simulink model "Single_String_with_shufflingconverters"  (R2019a)
settings: Solver=FixedStepDiscrete  StartTime=0.0  StopTime=0.2  RelTol=1e-3
libraries: powerlib x24, re_lib x4
settings Model: Creator=burge  LastModifiedBy=natha
settings DataIOCC: SaveState=on  ReturnWorkspaceOutputs=off
settings DebuggingCC: PregeneratedLibrarySubsystemCodeDiagnostic=none  ArithmeticOperatorsInVariantConditions=warning
settings SFSimCC: SimUseLocalCustomCode=off
settings RTWCC: RTWUseLocalCustomCode=off

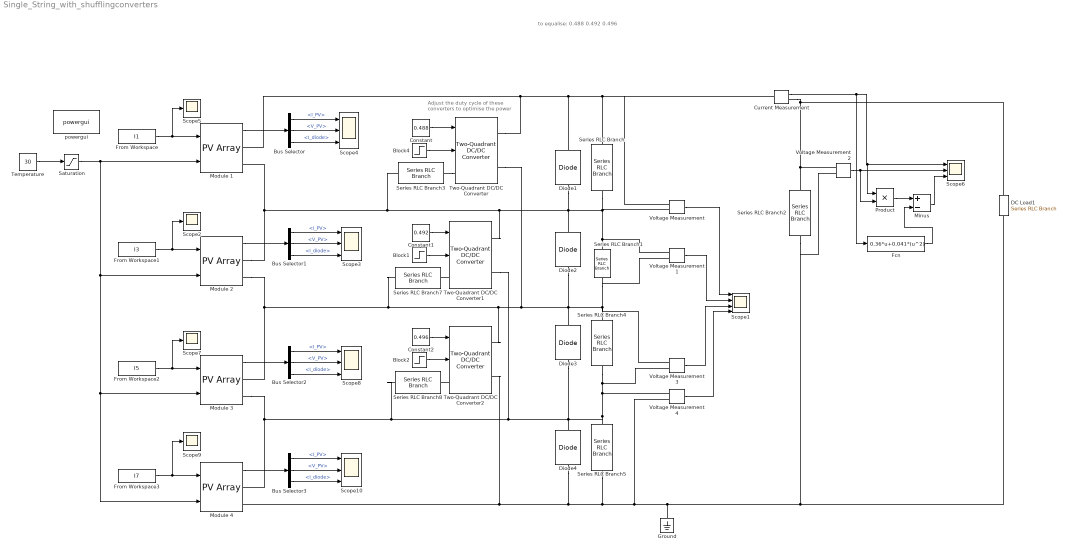
== system Single_String_with_shufflingconverters ==
  note: Adjust the duty cycle of these converters to optimise the power
  note: to equalise:
      | 0.488
      | 0.492
      | 0.496
  Block1 : Step  Time=0  Before=1  After=0  SampleTime=5e-5
  Block2 : Step  Time=0  Before=1  After=0  SampleTime=5e-5
  Block4 : Step  Time=0  Before=1  After=0  SampleTime=5e-5
  Bus Selector{,1..3} (4 alike) : BusSelector  OutputSignals=I_PV,V_PV,I_diode
  Constant : Constant  Value=0.488
  Constant1 : Constant  Value=0.492
  Constant2 : Constant  Value=0.496
  Current Measurement : powerlib/Measurements/Current Measurement  PhasorSimulation=off  OutputType=Complex  PSBequivalent=0
      settings: SourceProductName=Simscape Electrical
  DC Load1 : powerlib/Elements/Series RLC Branch  LConnTagsString=__new0  RConnTagsString=__new0  BranchType=R  Resistance=9  Inductance=1e-3  SetiL0=off  InitialCurrent=0  Capacitance=1e-6  Setx0=off  InitialVoltage=0  Measurements=None
      settings: SourceProductName=Simscape Electrical
  Diode{1..4} (4 alike) : powerlib/Power Electronics/Diode  Ron=0.05  Lon=0  Vf=0.7  IC=0  UseSnubber=0  Rs=500  Cs=250e-9  Measurements=off
      settings: SourceProductName=Simscape Electrical
  Fcn : Fcn  Expr=0.36*u+0.041*(u^2)
  From Workspace : FromWorkspace  VariableName=I1  OutDataTypeStr=double  SampleTime=0  OutputAfterFinalValue=Holding final value
  From Workspace1 : FromWorkspace  VariableName=I3  OutDataTypeStr=double  SampleTime=0  OutputAfterFinalValue=Holding final value
  From Workspace2 : FromWorkspace  VariableName=I5  OutDataTypeStr=double  SampleTime=0  OutputAfterFinalValue=Holding final value
  From Workspace3 : FromWorkspace  VariableName=I7  OutDataTypeStr=double  SampleTime=0  OutputAfterFinalValue=Holding final value
  Ground : powerlib/Elements/Ground  LConnTagsString=a
      settings: SourceProductName=Simscape Electrical
  Minus : Sum  Inputs=+-
  Module 1 : re_lib/Solar/PV Array  Npar=1  Nser=5  PlotType=array @ 1000 W/m2 & specified temperatures  S_vec="[ 1000  500  100 ]"  Temp_C_vec="[ 45 25  ]"  ModuleName=User-defined  PlotWhenSelected=off  Pm=3.8912  Ncell=1  Voc=0.727  Isc=6.45  Vm=0.64  Im=6.08  beta_Voc_pc=-0.2393  alpha_Isc_pc=0.045  beta_Voc=-0.0017397  alpha_Isc=0.0029025  IL=6.4807  I0=1.3352e-12  nI=0.96977  Rsh=3.547  Rs=0.00078547  BAL=on  Tc=1e-6  Tfilter=5e-5
      settings: SourceProductName=Simscape Electrical
  Module 2 : re_lib/Solar/PV Array  Npar=1  Nser=10  PlotType=array @ 1000 W/m2 & specified temperatures  S_vec="[ 1000  500  100 ]"  Temp_C_vec="[ 45 25  ]"  ModuleName=User-defined  PlotWhenSelected=off  Pm=3.8912  Ncell=1  Voc=0.727  Isc=6.45  Vm=0.64  Im=6.08  beta_Voc_pc=-0.2393  alpha_Isc_pc=0.045  beta_Voc=-0.0017397  alpha_Isc=0.0029025  IL=6.4807  I0=1.3352e-12  nI=0.96977  Rsh=3.547  Rs=0.00078547  BAL=on  Tc=1e-6  Tfilter=5e-5
      settings: SourceProductName=Simscape Electrical
  Module 3 : re_lib/Solar/PV Array  Npar=1  Nser=10  PlotType=array @ 1000 W/m2 & specified temperatures  S_vec="[ 1000  500  100 ]"  Temp_C_vec="[ 45 25  ]"  ModuleName=User-defined  PlotWhenSelected=off  Pm=3.8912  Ncell=1  Voc=0.727  Isc=6.45  Vm=0.64  Im=6.08  beta_Voc_pc=-0.2393  alpha_Isc_pc=0.045  beta_Voc=-0.0017397  alpha_Isc=0.0029025  IL=6.4807  I0=1.3352e-12  nI=0.96977  Rsh=3.547  Rs=0.00078547  BAL=on  Tc=1e-6  Tfilter=5e-5
      settings: SourceProductName=Simscape Electrical
  Module 4 : re_lib/Solar/PV Array  Npar=1  Nser=10  PlotType=array @ 1000 W/m2 & specified temperatures  S_vec="[ 1000  500  100 ]"  Temp_C_vec="[ 45 25  ]"  ModuleName=User-defined  PlotWhenSelected=off  Pm=3.8912  Ncell=1  Voc=0.727  Isc=6.45  Vm=0.64  Im=6.08  beta_Voc_pc=-0.2393  alpha_Isc_pc=0.045  beta_Voc=-0.0017397  alpha_Isc=0.0029025  IL=6.4807  I0=1.3352e-12  nI=0.96977  Rsh=3.547  Rs=0.00078547  BAL=on  Tc=1e-6  Tfilter=5e-5
      settings: SourceProductName=Simscape Electrical
  Product : Product
  Saturation : Saturate  UpperLimit=55  LowerLimit=5
  Scope1 : Scope  NumInputPorts=4
  Scope{3..4,6,8,10} (5 alike) : Scope  NumInputPorts=3
  Scope{2,5,7,9} (4 alike) : Scope
  Series RLC Branch{,1,4..5} (4 alike) : powerlib/Elements/Series RLC Branch  LConnTagsString=__new0  RConnTagsString=__new0  BranchType=C  Resistance=1  Inductance=1e-3  SetiL0=off  InitialCurrent=0  Capacitance=100e-6  Setx0=off  InitialVoltage=0  Measurements=None
      settings: SourceProductName=Simscape Electrical
  Series RLC Branch2 : powerlib/Elements/Series RLC Branch  LConnTagsString=__new0  RConnTagsString=__new0  BranchType=C  Resistance=1  Inductance=1e-3  SetiL0=off  InitialCurrent=0  Capacitance=10000e-6  Setx0=off  InitialVoltage=0  Measurements=None
      settings: SourceProductName=Simscape Electrical
  Series RLC Branch3 : powerlib/Elements/Series RLC Branch  LConnTagsString=__new0  RConnTagsString=__new0  BranchType=RL  Resistance=0.01  Inductance=1e-4  SetiL0=off  InitialCurrent=0  Capacitance=1e-6  Setx0=off  InitialVoltage=0  Measurements=None
      settings: SourceProductName=Simscape Electrical
  Series RLC Branch7 : powerlib/Elements/Series RLC Branch  LConnTagsString=__new0  RConnTagsString=__new0  BranchType=RL  Resistance=0.01  Inductance=1e-4  SetiL0=off  InitialCurrent=0  Capacitance=1e-6  Setx0=off  InitialVoltage=0  Measurements=None
      settings: SourceProductName=Simscape Electrical
  Series RLC Branch8 : powerlib/Elements/Series RLC Branch  LConnTagsString=__new0  RConnTagsString=__new0  BranchType=RL  Resistance=0.01  Inductance=1e-4  SetiL0=off  InitialCurrent=0  Capacitance=1e-6  Setx0=off  InitialVoltage=0  Measurements=None
      settings: SourceProductName=Simscape Electrical
  Temperature : Constant  Value=30
  Two-Quadrant DC/DC Converter : powerlib/Power Electronics/Two-Quadrant DC//DC Converter  ModelType=Average model (D-controlled)  Ron=1e-3  Rs=1e6  Cs=inf  Vforward=[0,0]  Ron_Diode=1e-3  Rs_Diode=1e6  Cs_Diode=inf  Vf_Diode=1e-3  Rs_CurrentSource=inf
      settings: SourceProductName=Simscape Electrical  SourceProductBaseCode=PS
  Two-Quadrant DC/DC Converter1 : powerlib/Power Electronics/Two-Quadrant DC//DC Converter  ModelType=Average model (D-controlled)  Ron=1e-3  Rs=1e6  Cs=inf  Vforward=[0,0]  Ron_Diode=1e-3  Rs_Diode=1e6  Cs_Diode=inf  Vf_Diode=1e-3  Rs_CurrentSource=inf
      settings: SourceProductName=Simscape Electrical  SourceProductBaseCode=PS
  Two-Quadrant DC/DC Converter2 : powerlib/Power Electronics/Two-Quadrant DC//DC Converter  ModelType=Average model (D-controlled)  Ron=1e-3  Rs=1e6  Cs=inf  Vforward=[0,0]  Ron_Diode=1e-3  Rs_Diode=1e6  Cs_Diode=inf  Vf_Diode=1e-3  Rs_CurrentSource=inf
      settings: SourceProductName=Simscape Electrical  SourceProductBaseCode=PS
  Voltage Measurement{,1..4} (5 alike) : powerlib/Measurements/Voltage Measurement  PhasorSimulation=off  OutputType=Complex  PSBequivalent=0
      settings: SourceProductName=Simscape Electrical
  powergui : powerlib/powergui  Priority=1  SimulationMode=Discrete  SampleTime=5e-6  frequency=60  Iterations=50  frequencyindice=0  Pbase=100e6  ErrMax=1e-4  UnitsV=kV  UnitsW=MW  buscounter=0  FunctionMessages=off  echomessages=off  EnableUseOfTLC=off  CurrentSourceSwitches=off  DisableSnubberDevices=off  DisableRonSwitches=off  DisableVfSwitches=off  DisplayEquations=off  AutomaticDiscreteSolvers=off  SolverType=Tustin/Backward Euler (TBE)  Interpol=off  ExternalGateDelay=off  methode=off  Ts=100  x0status=blocks  SPID=off  SwTol=0  HookPort=off  NonlinearTolerance=0  nMaxIteration=15  ContinueOnMaxIteration=off  RestoreLinks=warning  ResistiveCurrentMeasurement=off  Frange=[0:2:500]  Ylog=off  Xlog=on  ShowGrid=off  save=off  variable=ZData  structure=0  ZoomFFT=off  StartTime=0.0  cycles=1  DisplayStyle=1  fundamental=60  FreqAxis=off  MaxFrequency=1000  frequencyindicesteady=1  RmsSteady=1  display=off
      settings: SourceProductName=Simscape Electrical
  wires:
  Module 1/1 -> Bus Selector/1
  Bus Selector/1 -> Scope4/1  "<I_PV>"
  From Workspace/1 -> Scope5/1, Module 1/1
  Temperature/1 -> Saturation/1
  Bus Selector/2 -> Scope4/2  "<V_PV>"
  Bus Selector/3 -> Scope4/3  "<I_diode>"
  Voltage Measurement/1 -> Scope1/1
  Saturation/1 -> Module 4/2, Module 3/2, Module 2/2, Module 1/2
  From Workspace1/1 -> Scope2/1, Module 2/1
  Bus Selector1/2 -> Scope3/2  "<V_PV>"
  Bus Selector1/3 -> Scope3/3  "<I_diode>"
  Module 2/1 -> Bus Selector1/1
  Bus Selector1/1 -> Scope3/1  "<I_PV>"
  Voltage Measurement1/1 -> Scope1/2
  Voltage Measurement2/1 -> Product/2, Scope6/2
  Current Measurement/1 -> Fcn/1, Product/1, Scope6/1
  Constant/1 -> Two-Quadrant DC/DC Converter/1
  Block4/1 -> Two-Quadrant DC/DC Converter/2
  From Workspace2/1 -> Scope7/1, Module 3/1
  Bus Selector2/1 -> Scope8/1  "<I_PV>"
  Bus Selector2/3 -> Scope8/3  "<I_diode>"
  Bus Selector2/2 -> Scope8/2  "<V_PV>"
  Module 3/1 -> Bus Selector2/1
  Voltage Measurement3/1 -> Scope1/3
  From Workspace3/1 -> Scope9/1, Module 4/1
  Bus Selector3/2 -> Scope10/2  "<V_PV>"
  Bus Selector3/1 -> Scope10/1  "<I_PV>"
  Bus Selector3/3 -> Scope10/3  "<I_diode>"
  Module 4/1 -> Bus Selector3/1
  Voltage Measurement4/1 -> Scope1/4
  Block1/1 -> Two-Quadrant DC/DC Converter1/2
  Constant1/1 -> Two-Quadrant DC/DC Converter1/1
  Block2/1 -> Two-Quadrant DC/DC Converter2/2
  Constant2/1 -> Two-Quadrant DC/DC Converter2/1
  Fcn/1 -> Minus/2
  Minus/1 -> Scope6/3
  Product/1 -> Minus/1
  connections:
  Module 2/RConn1 -- Series RLC Branch3/LConn1 -- Two-Quadrant DC/DC Converter1/RConn1 -- Diode2/RConn1 -- Diode1/LConn1 -- Series RLC Branch/RConn1 -- Voltage Measurement/LConn2 -- Voltage Measurement1/LConn1 -- Series RLC Branch1/LConn1 -- Module 1/RConn2
  DC Load1/LConn1 -- Voltage Measurement2/LConn1 -- Series RLC Branch2/LConn1 -- Current Measurement/RConn1
  Series RLC Branch3/RConn1 -- Two-Quadrant DC/DC Converter/LConn1
  Module 2/RConn2 -- Module 3/RConn1 -- Series RLC Branch7/LConn1 -- Two-Quadrant DC/DC Converter2/RConn1 -- Two-Quadrant DC/DC Converter/RConn2 -- Diode2/LConn1 -- Voltage Measurement1/LConn2 -- Series RLC Branch1/RConn1 -- Voltage Measurement3/LConn1 -- Series RLC Branch4/LConn1 -- Diode3/RConn1
  Series RLC Branch4/RConn1 -- Voltage Measurement3/LConn2 -- Diode3/LConn1 -- Two-Quadrant DC/DC Converter1/RConn2 -- Series RLC Branch8/LConn1 -- Module 3/RConn2 -- Module 4/RConn1 -- Diode4/RConn1 -- Series RLC Branch5/LConn1 -- Voltage Measurement4/LConn1
  Series RLC Branch/LConn1 -- Current Measurement/LConn1 -- Voltage Measurement/LConn1 -- Two-Quadrant DC/DC Converter/RConn1 -- Module 1/RConn1 -- Diode1/RConn1
  Series RLC Branch7/RConn1 -- Two-Quadrant DC/DC Converter1/LConn1
  Series RLC Branch8/RConn1 -- Two-Quadrant DC/DC Converter2/LConn1
  Voltage Measurement2/LConn2 -- Series RLC Branch2/RConn1 -- DC Load1/RConn1 -- Ground/LConn1 -- Voltage Measurement4/LConn2 -- Diode4/LConn1 -- Two-Quadrant DC/DC Converter2/RConn2 -- Module 4/RConn2 -- Series RLC Branch5/RConn1
